simulink model "RHand_20DOF_Inv"  (R2020b)
settings: Solver=ode4  StartTime=0  StopTime=tTimeEnd  FixedStep=iStep  RelTol=1e-20  EnableMultiTasking=on
values from neighbouring files (symbols this model uses):
  g = 9.81    [getStaticTroques.m]    (also in ini_simbody_hand_19DOF.m; setModelParam_BoxSci.m)
  N = 18    [getStaticTroques.m]
undefined symbols (not defined in the file or in its folder): dof_mech_ra_cmc1_ad_ab, dof_mech_ra_cmc1_f_e, dof_mech_ra_dip2_e_f, dof_mech_ra_dip3_e_f, dof_mech_ra_dip4_e_f, dof_mech_ra_dip5_e_f, dof_mech_ra_el_e_f, dof_mech_ra_ip1_f_e, dof_mech_ra_mcp1_f_e, dof_mech_ra_mcp2_e_f, dof_mech_ra_mcp3_e_f, dof_mech_ra_mcp4_e_f, dof_mech_ra_mcp5_e_f, dof_mech_ra_pip2_e_f, dof_mech_ra_pip3_e_f, dof_mech_ra_pip4_e_f, dof_mech_ra_pip5_e_f, dof_mech_ra_wr_ad_ab, dof_mech_ra_wr_e_f, dof_mech_ra_wr_s_p, ic_ra_cmc1_ad_ab, ic_ra_cmc1_f_e, ic_ra_dip2_e_f, ic_ra_dip3_e_f, ic_ra_dip4_e_f, ic_ra_dip5_e_f, ic_ra_el_e_f, ic_ra_ip1_f_e, ic_ra_mcp1_f_e, ic_ra_mcp2_e_f, ic_ra_mcp3_e_f, ic_ra_mcp4_e_f, ic_ra_mcp5_e_f, ic_ra_pip2_e_f, ic_ra_pip3_e_f, ic_ra_pip4_e_f, ic_ra_pip5_e_f, ic_ra_wr_ad_ab, ic_ra_wr_e_f, ic_ra_wr_s_p, nScale, range_ra_cmc1_ad_ab, range_ra_cmc1_f_e, range_ra_dip2_e_f, range_ra_dip3_e_f, range_ra_dip4_e_f, range_ra_dip5_e_f, range_ra_el_e_f, range_ra_ip1_f_e, range_ra_mcp1_f_e, range_ra_mcp2_e_f, range_ra_mcp3_e_f, range_ra_mcp4_e_f, range_ra_mcp5_e_f, range_ra_pip2_e_f, range_ra_pip3_e_f, range_ra_pip4_e_f, range_ra_pip5_e_f, range_ra_wr_ad_ab, range_ra_wr_e_f ... (+4)
libraries: sm_lib x116, nesl_utility x41
(part 1 of 4)
settings Model: Creator=valeriya  LastModifiedBy=matthewyough
settings SolverCC: ShapePreserveControl=EnableAll  ZeroCrossControl=EnableAll  ZeroCrossAlgorithm=Adaptive  AutoInsertRateTranBlk=on
settings DataIOCC: SaveFormat=Array  SaveOutput=off  SignalLogging=off  DSMLogging=off  SaveTime=off  ReturnWorkspaceOutputs=off
settings OptimizationCC: LifeSpan=inf
settings DebuggingCC: InheritedTsInSrcMsg=none  SFUnexpectedBacktrackingDiag=warning  SFNoUnconditionalDefaultTransitionDiag=warning  SFExecutionAtInitializationDiag=none  ArithmeticOperatorsInVariantConditions=warning
settings HardwareCC: ProdBitPerPointer=32  ProdBitPerSizeT=32  ProdBitPerPtrDiffT=32  ProdLargestAtomicFloat=None  ProdIntDivRoundTo=Undefined  ProdEndianess=Unspecified  ProdWordSize=32  ProdHWDeviceType=32-bit Generic
settings ModelReferenceCC: PropagateSignalLabelsOutOfModel=off
settings SFSimCC: SimUseLocalCustomCode=off  CustomCodeUndefinedFunction=UseInterfaceOnly
settings RTWCC: RTWUseLocalCustomCode=off
settings CodeAppCC: StateflowObjectComments=on
settings GRTTargetCC: TargetLangStandard=C89/C90 (ANSI)
settings ConfigComp: CovMetricSettings=dw  CovSaveCumulativeToWorkspaceVar=on  CovSaveSingleToWorkspaceVar=on  CovExternalEMLEnable=off
settings SimscapeCC: SimscapeNormalizeSystem=off  SimscapeLogLimitData=off  SimscapeLogDataHistory=10000
settings ConfigurationSet: Description=SimMechanics 2G

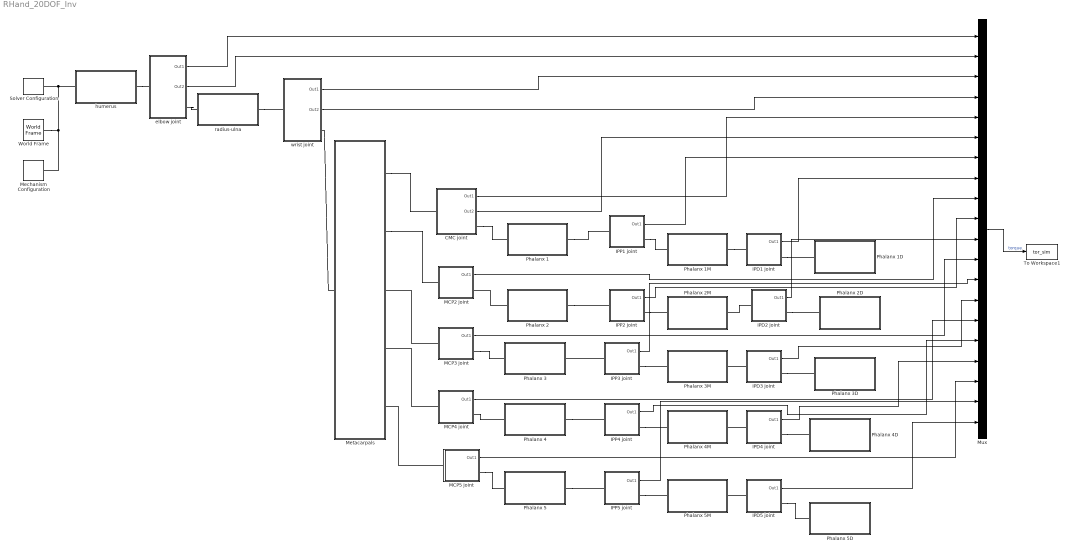
== system RHand_20DOF_Inv ==
  CMC joint : Subsystem
  IPD1 joint : Subsystem
  IPD2 joint : Subsystem
  IPD3 joint : Subsystem
  IPD4 joint : Subsystem
  IPD5 joint : Subsystem
  IPP1 joint : Subsystem
  IPP2 joint : Subsystem
  IPP3 joint : Subsystem
  IPP4 joint : Subsystem
  IPP5 joint : Subsystem
  MCP2 joint : Subsystem
  MCP3 joint : Subsystem
  MCP4 joint : Subsystem
  MCP5 joint : Subsystem
  Mechanism Configuration : sm_lib/Utilities/Mechanism Configuration  UniformGravity=Constant  GravityVector=[0 g 0]  GravityVectorUnits=m/s^2  GravityUnits=m/s^2  LinearizationDelta=0.000001  JointModeTransitionNonlinearIterations=2
  Metacarpals : Subsystem  mask{L=nScale.MC(1), W=nScale.MC(2), T=nScale.MC(3), CM=nScale.MC(4), M=nScale.MC(5)}
      mask prompts: L "Length (m)"; W "Width (m)"; T "Thickness (m)"; CM "Center of mass (m)"; M "Mass (kg)"
  Mux : Mux  Inputs=20
  Phalanx 1 : Subsystem  mask{L=nScale.P1(1), R=nScale.P1(2), CM=nScale.P1(4), M=nScale.P1(5)}
      mask prompts: L "Segment length (m)"; R "Segment radius (m)"; CM "Distance to the center of mass (m)"; M "Segment mass (kg)"
  Phalanx 1D : Subsystem  mask{L=nScale.P1D(1), R=nScale.P1D(2), CM=nScale.P1D(4), M=nScale.P1D(5)}
      mask prompts: L "Segment length (m)"; R "Segment radius (m)"; CM "Distance to the center of mass (m)"; M "Segment mass (kg)"
  Phalanx 1M : Subsystem  mask{L=nScale.P1M(1), R=nScale.P1M(2), CM=nScale.P1M(4), M=nScale.P1M(5)}
      mask prompts: L "Segment length (m)"; R "Segment radius (m)"; CM "Distance to the center of mass (m)"; M "Segment mass (kg)"
  Phalanx 2 : Subsystem  mask{L=nScale.P2(1), R=nScale.P2(2), CM=nScale.P2(4), M=nScale.P2(5)}
      mask prompts: L "Segment length (m)"; R "Segment radius (m)"; CM "Distance to the center of mass (m)"; M "Segment mass (kg)"
  Phalanx 2D : Subsystem  mask{L=nScale.P2D(1), R=nScale.P2D(2), CM=nScale.P2D(4), M=nScale.P2D(5)}
      mask prompts: L "Segment length (m)"; R "Segment radius (m)"; CM "Distance to the center of mass (m)"; M "Segment mass (kg)"
  Phalanx 2M : Subsystem  mask{L=nScale.P2M(1), R=nScale.P2M(2), CM=nScale.P2M(4), M=nScale.P2M(5)}
      mask prompts: L "Segment length (m)"; R "Segment radius (m)"; CM "Distance to the center of mass (m)"; M "Segment mass (kg)"
  Phalanx 3 : Subsystem  mask{L=nScale.P3(1), R=nScale.P3(2), CM=nScale.P3(4), M=nScale.P3(5)}
      mask prompts: L "Segment length (m)"; R "Segment radius (m)"; CM "Distance to the center of mass (m)"; M "Segment mass (kg)"
  Phalanx 3D : Subsystem  mask{L=nScale.P3D(1), R=nScale.P3D(2), CM=nScale.P3D(4), M=nScale.P3D(5)}
      mask prompts: L "Segment length (m)"; R "Segment radius (m)"; CM "Distance to the center of mass (m)"; M "Segment mass (kg)"
  Phalanx 3M : Subsystem  mask{L=nScale.P3M(1), R=nScale.P3M(2), CM=nScale.P3M(4), M=nScale.P3M(5)}
      mask prompts: L "Segment length (m)"; R "Segment radius (m)"; CM "Distance to the center of mass (m)"; M "Segment mass (kg)"
  Phalanx 4 : Subsystem  mask{L=nScale.P4(1), R=nScale.P4(2), CM=nScale.P4(4), M=nScale.P4(5)}
      mask prompts: L "Segment length (m)"; R "Segment radius (m)"; CM "Distance to the center of mass (m)"; M "Segment mass (kg)"
  Phalanx 4D : Subsystem  mask{L=nScale.P4D(1), R=nScale.P4D(2), CM=nScale.P4D(4), M=nScale.P4D(5)}
      mask prompts: L "Segment length (m)"; R "Segment radius (m)"; CM "Distance to the center of mass (m)"; M "Segment mass (kg)"
  Phalanx 4M : Subsystem  mask{L=nScale.P4M(1), R=nScale.P4M(2), CM=nScale.P4M(4), M=nScale.P4M(5)}
      mask prompts: L "Segment length (m)"; R "Segment radius (m)"; CM "Distance to the center of mass (m)"; M "Segment mass (kg)"
  Phalanx 5 : Subsystem  mask{L=nScale.P5(1), R=nScale.P5(2), CM=nScale.P5(4), M=nScale.P5(5)}
      mask prompts: L "Segment length (m)"; R "Segment radius (m)"; CM "Distance to the center of mass (m)"; M "Segment mass (kg)"
  Phalanx 5D : Subsystem  mask{L=nScale.P5D(1), R=nScale.P5D(2), CM=nScale.P5D(4), M=nScale.P5D(5)}
      mask prompts: L "Segment length (m)"; R "Segment radius (m)"; CM "Distance to the center of mass (m)"; M "Segment mass (kg)"
  Phalanx 5M : Subsystem  mask{L=nScale.P5M(1), R=nScale.P5M(2), CM=nScale.P5M(4), M=nScale.P5M(5)}
      mask prompts: L "Segment length (m)"; R "Segment radius (m)"; CM "Distance to the center of mass (m)"; M "Segment mass (kg)"
  Solver Configuration : nesl_utility/Solver Configuration  PhysicalDomain=network_engine_domain  SubClassName=solver  LeftPortType=input  RightPortType=generic  Tones=[]  Harmonics=[]  SimulateNoise=off  Profile=off  UseLocalSampling=off  EnableSwitchedLinearOptims=on  FrequencyDomain=off  UseCCode=off  RelTol=0.001  AbsTol=1e-06  MinStep=1e-09  ToWorkspace=off  RevertToSquareIcSolve=off  NumHomotopyIterations=100  PhasorMode=off  PhasorModeNumHarmonics=1  DoDC=on  ResidualTolerance=1e-48  UseLocalSolver=off  LocalSolverChoice=NE_BACKWARD_EULER_ADVANCER  LocalSolverSampleTime=iStep  DoFixedCost=off  MaxNonlinIter=3  MaxModeIter=2  ComputeImpulses=off  ImpulseIterations=2  LinearAlgebra=Full  EquationFormulation=NE_TIME_EF  DelaysMemoryBudget=1024  AutomaticFiltering=off  FilteringTimeConstant=0.01  PartitionStorageMethod=AS_NEEDED  PartitionMemoryBudget=1024  PartitionMethod=FAST
  To Workspace1 : ToWorkspace  VariableName=tor_sim  SaveFormat=Structure With Time  SampleTime=-1
  World Frame : sm_lib/Frames and Transforms/World Frame
  elbow joint : Subsystem
  humerus : Subsystem  mask{L=nScale.H(1), R=nScale.H(2), CM=nScale.H(4), M=nScale.H(5)}
      mask prompts: L "Segment length (m)"; R "Segment radius (m)"; CM "Distance to the center of mass (m)"; M "Segment mass (kg)"
  radius-ulna : Subsystem  mask{L=nScale.RU(1), R=nScale.RU(2), CM=nScale.RU(4), M=nScale.RU(5)}
      mask prompts: L "Segment length (m)"; R "Segment radius (m)"; CM "Distance to the center of mass (m)"; M "Segment mass (kg)"
  wrist joint : Subsystem
  wires:
  Mux/1 -> To Workspace1/1  "torque"
  elbow joint/1(Out1) -> Mux/1
  elbow joint/2(Out2) -> Mux/2
  wrist joint/2(Out2) -> Mux/4
  wrist joint/1(Out1) -> Mux/3
  CMC joint/1(Out1) -> Mux/5
  CMC joint/2(Out2) -> Mux/6
  IPP1 joint/1(Out1) -> Mux/7
  IPD1 joint/1(Out1) -> Mux/8
  IPD5 joint/1(Out1) -> Mux/20
  IPD2 joint/1(Out1) -> Mux/11
  IPP2 joint/1(Out1) -> Mux/10
  IPD3 joint/1(Out1) -> Mux/14
  IPD4 joint/1(Out1) -> Mux/17
  IPP5 joint/1(Out1) -> Mux/19
  IPP4 joint/1(Out1) -> Mux/16
  MCP5 joint/1(Out1) -> Mux/18
  MCP2 joint/1(Out1) -> Mux/9
  IPP3 joint/1(Out1) -> Mux/13
  MCP3 joint/1(Out1) -> Mux/12
  MCP4 joint/1(Out1) -> Mux/15
  connections:
  World Frame/RConn1 -- Solver Configuration/RConn1 -- humerus/LConn1 -- Mechanism Configuration/RConn1
  Metacarpals/LConn1 -- wrist joint/RConn1
  radius-ulna/RConn1 -- wrist joint/LConn1
  humerus/RConn1 -- elbow joint/LConn1
  elbow joint/RConn1 -- radius-ulna/LConn1
  Metacarpals/RConn1 -- CMC joint/LConn1
  CMC joint/RConn1 -- Phalanx 1/LConn1
  IPP1 joint/RConn1 -- Phalanx 1M/LConn1
  Phalanx 1/RConn1 -- IPP1 joint/LConn1
  IPD1 joint/RConn1 -- Phalanx 1D/LConn1
  Phalanx 1M/RConn1 -- IPD1 joint/LConn1
  IPP4 joint/RConn1 -- Phalanx 4M/LConn1
  Metacarpals/RConn2 -- MCP2 joint/LConn1
  Phalanx 4/RConn1 -- IPP4 joint/LConn1
  IPD4 joint/RConn1 -- Phalanx 4D/LConn1
  MCP4 joint/RConn1 -- Phalanx 4/LConn1
  IPD3 joint/LConn1 -- Phalanx 3M/RConn1
  Phalanx 2/RConn1 -- IPP2 joint/LConn1
  IPP3 joint/RConn1 -- Phalanx 3M/LConn1
  Phalanx 5/RConn1 -- IPP5 joint/LConn1
  IPD5 joint/LConn1 -- Phalanx 5M/RConn1
  IPD4 joint/LConn1 -- Phalanx 4M/RConn1
  IPP2 joint/RConn1 -- Phalanx 2M/LConn1
  MCP5 joint/RConn1 -- Phalanx 5/LConn1
  IPP3 joint/LConn1 -- Phalanx 3/RConn1
  IPD5 joint/RConn1 -- Phalanx 5D/LConn1
  Phalanx 2/LConn1 -- MCP2 joint/RConn1
  IPD2 joint/RConn1 -- Phalanx 2D/LConn1
  IPP5 joint/RConn1 -- Phalanx 5M/LConn1
  IPD2 joint/LConn1 -- Phalanx 2M/RConn1
  MCP3 joint/RConn1 -- Phalanx 3/LConn1
  IPD3 joint/RConn1 -- Phalanx 3D/LConn1
  MCP3 joint/LConn1 -- Metacarpals/RConn3
  MCP4 joint/LConn1 -- Metacarpals/RConn4
  MCP5 joint/LConn1 -- Metacarpals/RConn5

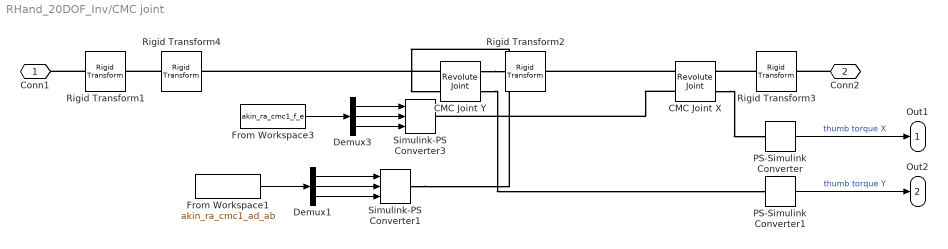
== system RHand_20DOF_Inv/CMC joint ==
  CMC Joint X : sm_lib/Joints/Revolute Joint  JointMode=Normal  SenseConstraintForce=off  SenseConstraintForceX=off  SenseConstraintForceY=off  SenseConstraintForceZ=off  SenseConstraintTorque=off  SenseConstraintTorqueX=off  SenseConstraintTorqueY=off  SenseConstraintTorqueZ=off  SenseTotalForce=off  SenseTotalForceX=off  SenseTotalForceY=off  SenseTotalForceZ=off  SenseTotalTorque=off  SenseTotalTorqueX=off  SenseTotalTorqueY=off  SenseTotalTorqueZ=off  CompositeWrenchDir=FollowerOnBase  CompositeWrenchFrame=BaseFrame  EquilibriumPosition=dof_mech_ra_cmc1_f_e(1)  EquilibriumPositionUnits=rad  SpringStiffness=dof_mech_ra_cmc1_f_e(2)  SpringStiffnessUnits=N*m/rad  DampingCoefficient=dof_mech_ra_cmc1_f_e(3)  DampingCoefficientUnits=N*m/(rad/s)  TorqueActuationMode=ComputedTorque  MotionActuationMode=InputMotion  SensePosition=off  SenseVelocity=off  SenseAcceleration=off  SenseTorqueForce=on  SenseLowerLimitTorqueForce=off  SenseUpperLimitTorqueForce=off  LowerLimitSpecify=on  LowerLimitBound=range_ra_cmc1_f_e(1)  LowerLimitBoundUnits=deg  LowerLimitStiffness=1e4  LowerLimitStiffnessUnits=N*m/deg  LowerLimitDamping=10  LowerLimitDampingUnits=N*m/(deg/s)  LowerLimitTransitionRegionWidth=0.1  LowerLimitTransitionRegionWidthUnits=deg  UpperLimitSpecify=on  UpperLimitBound=range_ra_cmc1_f_e(2)  UpperLimitBoundUnits=deg  UpperLimitStiffness=1e4  UpperLimitStiffnessUnits=N*m/deg  UpperLimitDamping=10  UpperLimitDampingUnits=N*m/(deg/s)  UpperLimitTransitionRegionWidth=0.1  UpperLimitTransitionRegionWidthUnits=deg  PositionTargetSpecify=off  PositionTargetPriority=High  PositionTargetValue=ic_ra_cmc1_f_e(1)  PositionTargetValueUnits=rad  VelocityTargetSpecify=off  VelocityTargetPriority=High  VelocityTargetValue=ic_ra_cmc1_f_e(2)  VelocityTargetValueUnits=rad/s
  CMC Joint Y : sm_lib/Joints/Revolute Joint  JointMode=Normal  SenseConstraintForce=off  SenseConstraintForceX=off  SenseConstraintForceY=off  SenseConstraintForceZ=off  SenseConstraintTorque=off  SenseConstraintTorqueX=off  SenseConstraintTorqueY=off  SenseConstraintTorqueZ=off  SenseTotalForce=off  SenseTotalForceX=off  SenseTotalForceY=off  SenseTotalForceZ=off  SenseTotalTorque=off  SenseTotalTorqueX=off  SenseTotalTorqueY=off  SenseTotalTorqueZ=off  CompositeWrenchDir=FollowerOnBase  CompositeWrenchFrame=BaseFrame  EquilibriumPosition=dof_mech_ra_cmc1_ad_ab(1)  EquilibriumPositionUnits=rad  SpringStiffness=dof_mech_ra_cmc1_ad_ab(2)  SpringStiffnessUnits=N*m/rad  DampingCoefficient=dof_mech_ra_cmc1_ad_ab(3)  DampingCoefficientUnits=N*m/(rad/s)  TorqueActuationMode=ComputedTorque  MotionActuationMode=InputMotion  SensePosition=off  SenseVelocity=off  SenseAcceleration=off  SenseTorqueForce=on  SenseLowerLimitTorqueForce=off  SenseUpperLimitTorqueForce=off  LowerLimitSpecify=on  LowerLimitBound=range_ra_cmc1_ad_ab(1)  LowerLimitBoundUnits=deg  LowerLimitStiffness=1e4  LowerLimitStiffnessUnits=N*m/deg  LowerLimitDamping=10  LowerLimitDampingUnits=N*m/(deg/s)  LowerLimitTransitionRegionWidth=0.1  LowerLimitTransitionRegionWidthUnits=deg  UpperLimitSpecify=on  UpperLimitBound=range_ra_cmc1_ad_ab(2)  UpperLimitBoundUnits=deg  UpperLimitStiffness=1e4  UpperLimitStiffnessUnits=N*m/deg  UpperLimitDamping=10  UpperLimitDampingUnits=N*m/(deg/s)  UpperLimitTransitionRegionWidth=0.1  UpperLimitTransitionRegionWidthUnits=deg  PositionTargetSpecify=off  PositionTargetPriority=High  PositionTargetValue=ic_ra_cmc1_ad_ab(1)  PositionTargetValueUnits=rad  VelocityTargetSpecify=off  VelocityTargetPriority=High  VelocityTargetValue=ic_ra_cmc1_ad_ab(2)  VelocityTargetValueUnits=rad/s
  Demux1 : Demux  Outputs=3
  Demux3 : Demux  Outputs=3
  From Workspace1 : FromWorkspace  VariableName=akin_ra_cmc1_ad_ab  SampleTime=-1  OutputAfterFinalValue=Holding final value
  From Workspace3 : FromWorkspace  VariableName=akin_ra_cmc1_f_e  SampleTime=-1  OutputAfterFinalValue=Holding final value
  PS-Simulink Converter : nesl_utility/PS-Simulink Converter  PhysicalDomain=network_engine_domain  SubClassName=ps_output  LeftPortType=input  RightPortType=output  PseudoPeriodic=off  Frequencies=[]  Unit=N*m  AffineConversion=off
  PS-Simulink Converter1 : nesl_utility/PS-Simulink Converter  PhysicalDomain=network_engine_domain  SubClassName=ps_output  LeftPortType=input  RightPortType=output  PseudoPeriodic=off  Frequencies=[]  Unit=N*m  AffineConversion=off
  Rigid Transform1 : sm_lib/Frames and Transforms/Rigid Transform  TranslationMethod=None  TranslationStandardOffset=0  TranslationLengthUnit=m  TranslationStandardAxis=+Z  TranslationCartesianOffset=[0 0 0]  TranslationROffset=0  TranslationROffsetUnits=m  TranslationZOffset=0  TranslationZOffsetUnits=m  TranslationThetaOffset=0  TranslationThetaOffsetUnits=deg  RotationMethod=StandardAxis  RotationAngleUnits=deg  RotationStandardAxis=-X  RotationAngle=180  RotationArbitraryAxis=[0 0 1]  FollAlignAxisA=+X  BaseAlignAxisA=+Y  FollAlignAxisB=+Y  BaseAlignAxisB=+Z  RotationSequenceAxes=FollowerAxes  RotationSequence=XYX  RotationSequenceAngles=[0 0 0]  RotationSequenceAnglesUnits=deg  RotationMatrix=[1 0 0; 0 1 0; 0 0 1]
  Rigid Transform2 : sm_lib/Frames and Transforms/Rigid Transform  TranslationMethod=None  TranslationStandardOffset=0  TranslationLengthUnit=m  TranslationStandardAxis=+Z  TranslationCartesianOffset=[0 0 0]  TranslationROffset=0  TranslationROffsetUnits=m  TranslationZOffset=0  TranslationZOffsetUnits=m  TranslationThetaOffset=0  TranslationThetaOffsetUnits=deg  RotationMethod=StandardAxis  RotationAngleUnits=deg  RotationStandardAxis=+Y  RotationAngle=90  RotationArbitraryAxis=[0 0 1]  FollAlignAxisA=+X  BaseAlignAxisA=+Y  FollAlignAxisB=+Y  BaseAlignAxisB=+Z  RotationSequenceAxes=FollowerAxes  RotationSequence=XYX  RotationSequenceAngles=[0 0 0]  RotationSequenceAnglesUnits=deg  RotationMatrix=[1 0 0; 0 1 0; 0 0 1]
  Rigid Transform3 : sm_lib/Frames and Transforms/Rigid Transform  TranslationMethod=None  TranslationStandardOffset=0  TranslationLengthUnit=m  TranslationStandardAxis=+Z  TranslationCartesianOffset=[0 0 0]  TranslationROffset=0  TranslationROffsetUnits=m  TranslationZOffset=0  TranslationZOffsetUnits=m  TranslationThetaOffset=0  TranslationThetaOffsetUnits=deg  RotationMethod=StandardAxis  RotationAngleUnits=deg  RotationStandardAxis=+X  RotationAngle=90  RotationArbitraryAxis=[0 0 1]  FollAlignAxisA=+X  BaseAlignAxisA=+Y  FollAlignAxisB=+Y  BaseAlignAxisB=+Z  RotationSequenceAxes=FollowerAxes  RotationSequence=XYX  RotationSequenceAngles=[0 0 0]  RotationSequenceAnglesUnits=deg  RotationMatrix=[1 0 0; 0 1 0; 0 0 1]
  Rigid Transform4 : sm_lib/Frames and Transforms/Rigid Transform  TranslationMethod=None  TranslationStandardOffset=0  TranslationLengthUnit=m  TranslationStandardAxis=+Z  TranslationCartesianOffset=[0 0 0]  TranslationROffset=0  TranslationROffsetUnits=m  TranslationZOffset=0  TranslationZOffsetUnits=m  TranslationThetaOffset=0  TranslationThetaOffsetUnits=deg  RotationMethod=StandardAxis  RotationAngleUnits=deg  RotationStandardAxis=+Y  RotationAngle=90  RotationArbitraryAxis=[0 0 1]  FollAlignAxisA=+X  BaseAlignAxisA=+Y  FollAlignAxisB=+Y  BaseAlignAxisB=+Z  RotationSequenceAxes=FollowerAxes  RotationSequence=XYX  RotationSequenceAngles=[0 0 0]  RotationSequenceAnglesUnits=deg  RotationMatrix=[1 0 0; 0 1 0; 0 0 1]
  Simulink-PS Converter1 : nesl_utility/Simulink-PS Converter  PhysicalDomain=network_engine_domain  SubClassName=ps_input  LeftPortType=input  RightPortType=output  PseudoPeriodic=off  Frequencies=[]  NoiseDistribution=none  NoiseParameters=[]  Unit=rad  AffineConversion=on  FilteringAndDerivatives=provide  SimscapeFilterOrder=2  InputFilterTimeConstant=0.001  UdotUserProvided=2
  Simulink-PS Converter3 : nesl_utility/Simulink-PS Converter  PhysicalDomain=network_engine_domain  SubClassName=ps_input  LeftPortType=input  RightPortType=output  PseudoPeriodic=off  Frequencies=[]  NoiseDistribution=none  NoiseParameters=[]  Unit=rad  AffineConversion=on  FilteringAndDerivatives=provide  SimscapeFilterOrder=2  InputFilterTimeConstant=0.001  UdotUserProvided=2
  Conn1 : PMIOPort  Side=Left
  Conn2 : PMIOPort  Port=2  Side=Right
  Out1 : Outport  VectorParamsAs1DForOutWhenUnconnected=off
  Out2 : Outport  Port=2  VectorParamsAs1DForOutWhenUnconnected=off
  wires:
  Demux3/1 -> Simulink-PS Converter3/1
  From Workspace3/1 -> Demux3/1
  Demux3/3 -> Simulink-PS Converter3/3
  Demux3/2 -> Simulink-PS Converter3/2
  Demux1/1 -> Simulink-PS Converter1/1
  From Workspace1/1 -> Demux1/1
  Demux1/3 -> Simulink-PS Converter1/3
  Demux1/2 -> Simulink-PS Converter1/2
  PS-Simulink Converter/1 -> Out1/1  "thumb torque X"
  PS-Simulink Converter1/1 -> Out2/1  "thumb torque Y"
  connections:
  CMC Joint X/LConn2 -- Simulink-PS Converter3/RConn1
  CMC Joint X/RConn2 -- PS-Simulink Converter/LConn1
  Rigid Transform1/LConn1 -- Conn1/RConn1
  CMC Joint Y/LConn1 -- Rigid Transform4/RConn1
  Simulink-PS Converter1/RConn1 -- CMC Joint Y/LConn2
  CMC Joint Y/RConn2 -- PS-Simulink Converter1/LConn1
  CMC Joint Y/RConn1 -- Rigid Transform2/LConn1
  CMC Joint X/LConn1 -- Rigid Transform2/RConn1
  Conn2/RConn1 -- Rigid Transform3/RConn1
  Rigid Transform4/LConn1 -- Rigid Transform1/RConn1
  Rigid Transform3/LConn1 -- CMC Joint X/RConn1

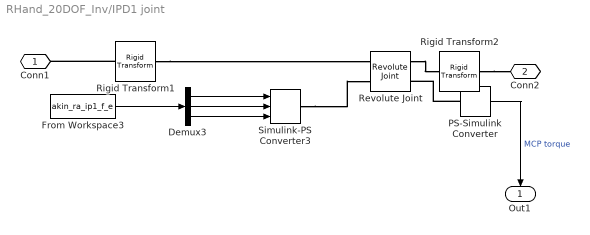
== system RHand_20DOF_Inv/IPD1 joint ==
  Demux3 : Demux  Outputs=3
  From Workspace3 : FromWorkspace  VariableName=akin_ra_ip1_f_e  SampleTime=-1  OutputAfterFinalValue=Holding final value
  PS-Simulink Converter : nesl_utility/PS-Simulink Converter  PhysicalDomain=network_engine_domain  SubClassName=ps_output  LeftPortType=input  RightPortType=output  PseudoPeriodic=off  Frequencies=[]  Unit=N*m  AffineConversion=off
  Revolute Joint : sm_lib/Joints/Revolute Joint  JointMode=Normal  SenseConstraintForce=off  SenseConstraintForceX=off  SenseConstraintForceY=off  SenseConstraintForceZ=off  SenseConstraintTorque=off  SenseConstraintTorqueX=off  SenseConstraintTorqueY=off  SenseConstraintTorqueZ=off  SenseTotalForce=off  SenseTotalForceX=off  SenseTotalForceY=off  SenseTotalForceZ=off  SenseTotalTorque=off  SenseTotalTorqueX=off  SenseTotalTorqueY=off  SenseTotalTorqueZ=off  CompositeWrenchDir=FollowerOnBase  CompositeWrenchFrame=BaseFrame  EquilibriumPosition=dof_mech_ra_ip1_f_e(1)  EquilibriumPositionUnits=rad  SpringStiffness=dof_mech_ra_ip1_f_e(2)  SpringStiffnessUnits=N*m/rad  DampingCoefficient=dof_mech_ra_ip1_f_e(3)  DampingCoefficientUnits=N*m/(rad/s)  TorqueActuationMode=ComputedTorque  MotionActuationMode=InputMotion  SensePosition=off  SenseVelocity=off  SenseAcceleration=off  SenseTorqueForce=on  SenseLowerLimitTorqueForce=off  SenseUpperLimitTorqueForce=off  LowerLimitSpecify=on  LowerLimitBound=range_ra_ip1_f_e(1)  LowerLimitBoundUnits=deg  LowerLimitStiffness=1e4  LowerLimitStiffnessUnits=N*m/deg  LowerLimitDamping=10  LowerLimitDampingUnits=N*m/(deg/s)  LowerLimitTransitionRegionWidth=0.1  LowerLimitTransitionRegionWidthUnits=deg  UpperLimitSpecify=on  UpperLimitBound=range_ra_ip1_f_e(2)  UpperLimitBoundUnits=deg  UpperLimitStiffness=1e4  UpperLimitStiffnessUnits=N*m/deg  UpperLimitDamping=10  UpperLimitDampingUnits=N*m/(deg/s)  UpperLimitTransitionRegionWidth=0.1  UpperLimitTransitionRegionWidthUnits=deg  PositionTargetSpecify=off  PositionTargetPriority=High  PositionTargetValue=ic_ra_ip1_f_e(1)  PositionTargetValueUnits=rad  VelocityTargetSpecify=off  VelocityTargetPriority=High  VelocityTargetValue=ic_ra_ip1_f_e(2)  VelocityTargetValueUnits=rad/s
  Rigid Transform1 : sm_lib/Frames and Transforms/Rigid Transform  TranslationMethod=None  TranslationStandardOffset=0  TranslationLengthUnit=m  TranslationStandardAxis=+Z  TranslationCartesianOffset=[0 0 0]  TranslationROffset=0  TranslationROffsetUnits=m  TranslationZOffset=0  TranslationZOffsetUnits=m  TranslationThetaOffset=0  TranslationThetaOffsetUnits=deg  RotationMethod=StandardAxis  RotationAngleUnits=deg  RotationStandardAxis=-X  RotationAngle=90  RotationArbitraryAxis=[0 0 1]  FollAlignAxisA=+X  BaseAlignAxisA=+Y  FollAlignAxisB=+Y  BaseAlignAxisB=+Z  RotationSequenceAxes=FollowerAxes  RotationSequence=XYX  RotationSequenceAngles=[0 0 0]  RotationSequenceAnglesUnits=deg  RotationMatrix=[1 0 0; 0 1 0; 0 0 1]
  Rigid Transform2 : sm_lib/Frames and Transforms/Rigid Transform  TranslationMethod=None  TranslationStandardOffset=0  TranslationLengthUnit=m  TranslationStandardAxis=+Z  TranslationCartesianOffset=[0 0 0]  TranslationROffset=0  TranslationROffsetUnits=m  TranslationZOffset=0  TranslationZOffsetUnits=m  TranslationThetaOffset=0  TranslationThetaOffsetUnits=deg  RotationMethod=StandardAxis  RotationAngleUnits=deg  RotationStandardAxis=+X  RotationAngle=90  RotationArbitraryAxis=[0 0 1]  FollAlignAxisA=+X  BaseAlignAxisA=+Y  FollAlignAxisB=+Y  BaseAlignAxisB=+Z  RotationSequenceAxes=FollowerAxes  RotationSequence=XYX  RotationSequenceAngles=[0 0 0]  RotationSequenceAnglesUnits=deg  RotationMatrix=[1 0 0; 0 1 0; 0 0 1]
  Simulink-PS Converter3 : nesl_utility/Simulink-PS Converter  PhysicalDomain=network_engine_domain  SubClassName=ps_input  LeftPortType=input  RightPortType=output  PseudoPeriodic=off  Frequencies=[]  NoiseDistribution=none  NoiseParameters=[]  Unit=rad  AffineConversion=on  FilteringAndDerivatives=provide  SimscapeFilterOrder=2  InputFilterTimeConstant=0.001  UdotUserProvided=2
  Conn1 : PMIOPort  Side=Left
  Conn2 : PMIOPort  Port=2  Side=Right
  Out1 : Outport  VectorParamsAs1DForOutWhenUnconnected=off
  wires:
  Demux3/1 -> Simulink-PS Converter3/1
  From Workspace3/1 -> Demux3/1
  Demux3/3 -> Simulink-PS Converter3/3
  PS-Simulink Converter/1 -> Out1/1  "MCP torque"
  Demux3/2 -> Simulink-PS Converter3/2
  connections:
  Simulink-PS Converter3/RConn1 -- Revolute Joint/LConn2
  PS-Simulink Converter/LConn1 -- Revolute Joint/RConn2
  Revolute Joint/RConn1 -- Rigid Transform2/LConn1
  Rigid Transform1/LConn1 -- Conn1/RConn1
  Rigid Transform1/RConn1 -- Revolute Joint/LConn1
  Rigid Transform2/RConn1 -- Conn2/RConn1

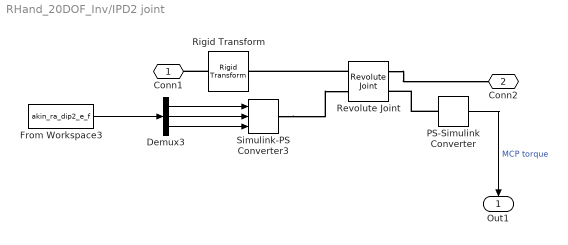
== system RHand_20DOF_Inv/IPD2 joint ==
  Demux3 : Demux  Outputs=3
  From Workspace3 : FromWorkspace  VariableName=akin_ra_dip2_e_f  SampleTime=-1  OutputAfterFinalValue=Holding final value
  PS-Simulink Converter : nesl_utility/PS-Simulink Converter  PhysicalDomain=network_engine_domain  SubClassName=ps_output  LeftPortType=input  RightPortType=output  PseudoPeriodic=off  Frequencies=[]  Unit=N*m  AffineConversion=off
  Revolute Joint : sm_lib/Joints/Revolute Joint  JointMode=Normal  SenseConstraintForce=off  SenseConstraintForceX=off  SenseConstraintForceY=off  SenseConstraintForceZ=off  SenseConstraintTorque=off  SenseConstraintTorqueX=off  SenseConstraintTorqueY=off  SenseConstraintTorqueZ=off  SenseTotalForce=off  SenseTotalForceX=off  SenseTotalForceY=off  SenseTotalForceZ=off  SenseTotalTorque=off  SenseTotalTorqueX=off  SenseTotalTorqueY=off  SenseTotalTorqueZ=off  CompositeWrenchDir=FollowerOnBase  CompositeWrenchFrame=BaseFrame  EquilibriumPosition=dof_mech_ra_dip2_e_f(1)  EquilibriumPositionUnits=rad  SpringStiffness=dof_mech_ra_dip2_e_f(2)  SpringStiffnessUnits=N*m/rad  DampingCoefficient=dof_mech_ra_dip2_e_f(3)  DampingCoefficientUnits=N*m/(rad/s)  TorqueActuationMode=ComputedTorque  MotionActuationMode=InputMotion  SensePosition=off  SenseVelocity=off  SenseAcceleration=off  SenseTorqueForce=on  SenseLowerLimitTorqueForce=off  SenseUpperLimitTorqueForce=off  LowerLimitSpecify=on  LowerLimitBound=range_ra_dip2_e_f(1)  LowerLimitBoundUnits=deg  LowerLimitStiffness=1e4  LowerLimitStiffnessUnits=N*m/deg  LowerLimitDamping=10  LowerLimitDampingUnits=N*m/(deg/s)  LowerLimitTransitionRegionWidth=0.1  LowerLimitTransitionRegionWidthUnits=deg  UpperLimitSpecify=on  UpperLimitBound=range_ra_dip2_e_f(2)  UpperLimitBoundUnits=deg  UpperLimitStiffness=1e4  UpperLimitStiffnessUnits=N*m/deg  UpperLimitDamping=10  UpperLimitDampingUnits=N*m/(deg/s)  UpperLimitTransitionRegionWidth=0.1  UpperLimitTransitionRegionWidthUnits=deg  PositionTargetSpecify=off  PositionTargetPriority=High  PositionTargetValue=ic_ra_dip2_e_f(1)  PositionTargetValueUnits=rad  VelocityTargetSpecify=off  VelocityTargetPriority=High  VelocityTargetValue=ic_ra_dip2_e_f(2)  VelocityTargetValueUnits=rad/s
  Rigid Transform : sm_lib/Frames and Transforms/Rigid Transform  TranslationMethod=None  TranslationStandardOffset=0  TranslationLengthUnit=m  TranslationStandardAxis=+Z  TranslationCartesianOffset=[0 0 0]  TranslationROffset=0  TranslationROffsetUnits=m  TranslationZOffset=0  TranslationZOffsetUnits=m  TranslationThetaOffset=0  TranslationThetaOffsetUnits=deg  RotationMethod=StandardAxis  RotationAngleUnits=deg  RotationStandardAxis=-Z  RotationAngle=180  RotationArbitraryAxis=[0 0 1]  FollAlignAxisA=+X  BaseAlignAxisA=+Y  FollAlignAxisB=+Y  BaseAlignAxisB=+Z  RotationSequenceAxes=FollowerAxes  RotationSequence=XYX  RotationSequenceAngles=[0 0 0]  RotationSequenceAnglesUnits=deg  RotationMatrix=[1 0 0; 0 1 0; 0 0 1]
  Simulink-PS Converter3 : nesl_utility/Simulink-PS Converter  PhysicalDomain=network_engine_domain  SubClassName=ps_input  LeftPortType=input  RightPortType=output  PseudoPeriodic=off  Frequencies=[]  NoiseDistribution=none  NoiseParameters=[]  Unit=rad  AffineConversion=on  FilteringAndDerivatives=provide  SimscapeFilterOrder=2  InputFilterTimeConstant=0.001  UdotUserProvided=2
  Conn1 : PMIOPort  Side=Left
  Conn2 : PMIOPort  Port=2  Side=Right
  Out1 : Outport  VectorParamsAs1DForOutWhenUnconnected=off
  wires:
  Demux3/1 -> Simulink-PS Converter3/1
  From Workspace3/1 -> Demux3/1
  Demux3/3 -> Simulink-PS Converter3/3
  PS-Simulink Converter/1 -> Out1/1  "MCP torque"
  Demux3/2 -> Simulink-PS Converter3/2
  connections:
  Simulink-PS Converter3/RConn1 -- Revolute Joint/LConn2
  PS-Simulink Converter/LConn1 -- Revolute Joint/RConn2
  Revolute Joint/RConn1 -- Conn2/RConn1
  Revolute Joint/LConn1 -- Rigid Transform/RConn1
  Rigid Transform/LConn1 -- Conn1/RConn1

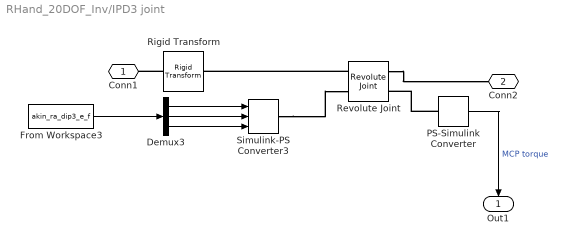
== system RHand_20DOF_Inv/IPD3 joint ==
  Demux3 : Demux  Outputs=3
  From Workspace3 : FromWorkspace  VariableName=akin_ra_dip3_e_f  SampleTime=-1  OutputAfterFinalValue=Holding final value
  PS-Simulink Converter : nesl_utility/PS-Simulink Converter  PhysicalDomain=network_engine_domain  SubClassName=ps_output  LeftPortType=input  RightPortType=output  PseudoPeriodic=off  Frequencies=[]  Unit=N*m  AffineConversion=off
  Revolute Joint : sm_lib/Joints/Revolute Joint  JointMode=Normal  SenseConstraintForce=off  SenseConstraintForceX=off  SenseConstraintForceY=off  SenseConstraintForceZ=off  SenseConstraintTorque=off  SenseConstraintTorqueX=off  SenseConstraintTorqueY=off  SenseConstraintTorqueZ=off  SenseTotalForce=off  SenseTotalForceX=off  SenseTotalForceY=off  SenseTotalForceZ=off  SenseTotalTorque=off  SenseTotalTorqueX=off  SenseTotalTorqueY=off  SenseTotalTorqueZ=off  CompositeWrenchDir=FollowerOnBase  CompositeWrenchFrame=BaseFrame  EquilibriumPosition=dof_mech_ra_dip3_e_f(1)  EquilibriumPositionUnits=rad  SpringStiffness=dof_mech_ra_dip3_e_f(2)  SpringStiffnessUnits=N*m/rad  DampingCoefficient=dof_mech_ra_dip3_e_f(3)  DampingCoefficientUnits=N*m/(rad/s)  TorqueActuationMode=ComputedTorque  MotionActuationMode=InputMotion  SensePosition=off  SenseVelocity=off  SenseAcceleration=off  SenseTorqueForce=on  SenseLowerLimitTorqueForce=off  SenseUpperLimitTorqueForce=off  LowerLimitSpecify=on  LowerLimitBound=range_ra_dip3_e_f(1)  LowerLimitBoundUnits=deg  LowerLimitStiffness=1e4  LowerLimitStiffnessUnits=N*m/deg  LowerLimitDamping=10  LowerLimitDampingUnits=N*m/(deg/s)  LowerLimitTransitionRegionWidth=0.1  LowerLimitTransitionRegionWidthUnits=deg  UpperLimitSpecify=on  UpperLimitBound=range_ra_dip3_e_f(2)  UpperLimitBoundUnits=deg  UpperLimitStiffness=1e4  UpperLimitStiffnessUnits=N*m/deg  UpperLimitDamping=10  UpperLimitDampingUnits=N*m/(deg/s)  UpperLimitTransitionRegionWidth=0.1  UpperLimitTransitionRegionWidthUnits=deg  PositionTargetSpecify=on  PositionTargetPriority=High  PositionTargetValue=ic_ra_dip3_e_f(1)  PositionTargetValueUnits=rad  VelocityTargetSpecify=on  VelocityTargetPriority=High  VelocityTargetValue=ic_ra_dip3_e_f(2)  VelocityTargetValueUnits=rad/s
  Rigid Transform : sm_lib/Frames and Transforms/Rigid Transform  TranslationMethod=None  TranslationStandardOffset=0  TranslationLengthUnit=m  TranslationStandardAxis=+Z  TranslationCartesianOffset=[0 0 0]  TranslationROffset=0  TranslationROffsetUnits=m  TranslationZOffset=0  TranslationZOffsetUnits=m  TranslationThetaOffset=0  TranslationThetaOffsetUnits=deg  RotationMethod=StandardAxis  RotationAngleUnits=deg  RotationStandardAxis=-Z  RotationAngle=180  RotationArbitraryAxis=[0 0 1]  FollAlignAxisA=+X  BaseAlignAxisA=+Y  FollAlignAxisB=+Y  BaseAlignAxisB=+Z  RotationSequenceAxes=FollowerAxes  RotationSequence=XYX  RotationSequenceAngles=[0 0 0]  RotationSequenceAnglesUnits=deg  RotationMatrix=[1 0 0; 0 1 0; 0 0 1]
  Simulink-PS Converter3 : nesl_utility/Simulink-PS Converter  PhysicalDomain=network_engine_domain  SubClassName=ps_input  LeftPortType=input  RightPortType=output  PseudoPeriodic=off  Frequencies=[]  NoiseDistribution=none  NoiseParameters=[]  Unit=rad  AffineConversion=on  FilteringAndDerivatives=provide  SimscapeFilterOrder=2  InputFilterTimeConstant=0.001  UdotUserProvided=2
  Conn1 : PMIOPort  Side=Left
  Conn2 : PMIOPort  Port=2  Side=Right
  Out1 : Outport  VectorParamsAs1DForOutWhenUnconnected=off
  wires:
  Demux3/1 -> Simulink-PS Converter3/1
  From Workspace3/1 -> Demux3/1
  Demux3/3 -> Simulink-PS Converter3/3
  PS-Simulink Converter/1 -> Out1/1  "MCP torque"
  Demux3/2 -> Simulink-PS Converter3/2
  connections:
  Simulink-PS Converter3/RConn1 -- Revolute Joint/LConn2
  PS-Simulink Converter/LConn1 -- Revolute Joint/RConn2
  Revolute Joint/RConn1 -- Conn2/RConn1
  Rigid Transform/LConn1 -- Conn1/RConn1
  Revolute Joint/LConn1 -- Rigid Transform/RConn1

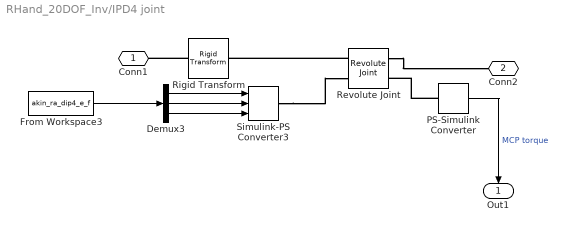
== system RHand_20DOF_Inv/IPD4 joint ==
  Demux3 : Demux  Outputs=3
  From Workspace3 : FromWorkspace  VariableName=akin_ra_dip4_e_f  SampleTime=-1  OutputAfterFinalValue=Holding final value
  PS-Simulink Converter : nesl_utility/PS-Simulink Converter  PhysicalDomain=network_engine_domain  SubClassName=ps_output  LeftPortType=input  RightPortType=output  PseudoPeriodic=off  Frequencies=[]  Unit=N*m  AffineConversion=off
  Revolute Joint : sm_lib/Joints/Revolute Joint  JointMode=Normal  SenseConstraintForce=off  SenseConstraintForceX=off  SenseConstraintForceY=off  SenseConstraintForceZ=off  SenseConstraintTorque=off  SenseConstraintTorqueX=off  SenseConstraintTorqueY=off  SenseConstraintTorqueZ=off  SenseTotalForce=off  SenseTotalForceX=off  SenseTotalForceY=off  SenseTotalForceZ=off  SenseTotalTorque=off  SenseTotalTorqueX=off  SenseTotalTorqueY=off  SenseTotalTorqueZ=off  CompositeWrenchDir=FollowerOnBase  CompositeWrenchFrame=BaseFrame  EquilibriumPosition=dof_mech_ra_dip4_e_f(1)  EquilibriumPositionUnits=rad  SpringStiffness=dof_mech_ra_dip4_e_f(2)  SpringStiffnessUnits=N*m/rad  DampingCoefficient=dof_mech_ra_dip4_e_f(3)  DampingCoefficientUnits=N*m/(rad/s)  TorqueActuationMode=ComputedTorque  MotionActuationMode=InputMotion  SensePosition=off  SenseVelocity=off  SenseAcceleration=off  SenseTorqueForce=on  SenseLowerLimitTorqueForce=off  SenseUpperLimitTorqueForce=off  LowerLimitSpecify=on  LowerLimitBound=range_ra_dip4_e_f(1)  LowerLimitBoundUnits=deg  LowerLimitStiffness=1e4  LowerLimitStiffnessUnits=N*m/deg  LowerLimitDamping=10  LowerLimitDampingUnits=N*m/(deg/s)  LowerLimitTransitionRegionWidth=0.1  LowerLimitTransitionRegionWidthUnits=deg  UpperLimitSpecify=on  UpperLimitBound=range_ra_dip4_e_f(2)  UpperLimitBoundUnits=deg  UpperLimitStiffness=1e4  UpperLimitStiffnessUnits=N*m/deg  UpperLimitDamping=10  UpperLimitDampingUnits=N*m/(deg/s)  UpperLimitTransitionRegionWidth=0.1  UpperLimitTransitionRegionWidthUnits=deg  PositionTargetSpecify=off  PositionTargetPriority=High  PositionTargetValue=ic_ra_dip4_e_f(1)  PositionTargetValueUnits=rad  VelocityTargetSpecify=off  VelocityTargetPriority=High  VelocityTargetValue=ic_ra_dip4_e_f(2)  VelocityTargetValueUnits=rad/s
  Rigid Transform : sm_lib/Frames and Transforms/Rigid Transform  TranslationMethod=None  TranslationStandardOffset=0  TranslationLengthUnit=m  TranslationStandardAxis=+Z  TranslationCartesianOffset=[0 0 0]  TranslationROffset=0  TranslationROffsetUnits=m  TranslationZOffset=0  TranslationZOffsetUnits=m  TranslationThetaOffset=0  TranslationThetaOffsetUnits=deg  RotationMethod=StandardAxis  RotationAngleUnits=deg  RotationStandardAxis=-Z  RotationAngle=180  RotationArbitraryAxis=[0 0 1]  FollAlignAxisA=+X  BaseAlignAxisA=+Y  FollAlignAxisB=+Y  BaseAlignAxisB=+Z  RotationSequenceAxes=FollowerAxes  RotationSequence=XYX  RotationSequenceAngles=[0 0 0]  RotationSequenceAnglesUnits=deg  RotationMatrix=[1 0 0; 0 1 0; 0 0 1]
  Simulink-PS Converter3 : nesl_utility/Simulink-PS Converter  PhysicalDomain=network_engine_domain  SubClassName=ps_input  LeftPortType=input  RightPortType=output  PseudoPeriodic=off  Frequencies=[]  NoiseDistribution=none  NoiseParameters=[]  Unit=rad  AffineConversion=on  FilteringAndDerivatives=provide  SimscapeFilterOrder=2  InputFilterTimeConstant=0.001  UdotUserProvided=2
  Conn1 : PMIOPort  Side=Left
  Conn2 : PMIOPort  Port=2  Side=Right
  Out1 : Outport  VectorParamsAs1DForOutWhenUnconnected=off
  wires:
  Demux3/1 -> Simulink-PS Converter3/1
  From Workspace3/1 -> Demux3/1
  Demux3/3 -> Simulink-PS Converter3/3
  PS-Simulink Converter/1 -> Out1/1  "MCP torque"
  Demux3/2 -> Simulink-PS Converter3/2
  connections:
  Simulink-PS Converter3/RConn1 -- Revolute Joint/LConn2
  PS-Simulink Converter/LConn1 -- Revolute Joint/RConn2
  Revolute Joint/RConn1 -- Conn2/RConn1
  Rigid Transform/LConn1 -- Conn1/RConn1
  Revolute Joint/LConn1 -- Rigid Transform/RConn1

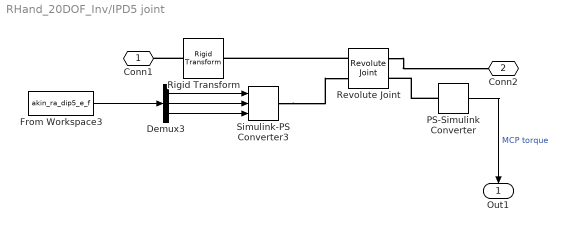
== system RHand_20DOF_Inv/IPD5 joint ==
  Demux3 : Demux  Outputs=3
  From Workspace3 : FromWorkspace  VariableName=akin_ra_dip5_e_f  SampleTime=-1  OutputAfterFinalValue=Holding final value
  PS-Simulink Converter : nesl_utility/PS-Simulink Converter  PhysicalDomain=network_engine_domain  SubClassName=ps_output  LeftPortType=input  RightPortType=output  PseudoPeriodic=off  Frequencies=[]  Unit=N*m  AffineConversion=off
  Revolute Joint : sm_lib/Joints/Revolute Joint  JointMode=Normal  SenseConstraintForce=off  SenseConstraintForceX=off  SenseConstraintForceY=off  SenseConstraintForceZ=off  SenseConstraintTorque=off  SenseConstraintTorqueX=off  SenseConstraintTorqueY=off  SenseConstraintTorqueZ=off  SenseTotalForce=off  SenseTotalForceX=off  SenseTotalForceY=off  SenseTotalForceZ=off  SenseTotalTorque=off  SenseTotalTorqueX=off  SenseTotalTorqueY=off  SenseTotalTorqueZ=off  CompositeWrenchDir=FollowerOnBase  CompositeWrenchFrame=BaseFrame  EquilibriumPosition=dof_mech_ra_dip5_e_f(1)  EquilibriumPositionUnits=rad  SpringStiffness=dof_mech_ra_dip5_e_f(2)  SpringStiffnessUnits=N*m/rad  DampingCoefficient=dof_mech_ra_dip5_e_f(3)  DampingCoefficientUnits=N*m/(rad/s)  TorqueActuationMode=ComputedTorque  MotionActuationMode=InputMotion  SensePosition=off  SenseVelocity=off  SenseAcceleration=off  SenseTorqueForce=on  SenseLowerLimitTorqueForce=off  SenseUpperLimitTorqueForce=off  LowerLimitSpecify=on  LowerLimitBound=range_ra_dip5_e_f(1)  LowerLimitBoundUnits=deg  LowerLimitStiffness=1e4  LowerLimitStiffnessUnits=N*m/deg  LowerLimitDamping=10  LowerLimitDampingUnits=N*m/(deg/s)  LowerLimitTransitionRegionWidth=0.1  LowerLimitTransitionRegionWidthUnits=deg  UpperLimitSpecify=on  UpperLimitBound=range_ra_dip5_e_f(2)  UpperLimitBoundUnits=deg  UpperLimitStiffness=1e4  UpperLimitStiffnessUnits=N*m/deg  UpperLimitDamping=10  UpperLimitDampingUnits=N*m/(deg/s)  UpperLimitTransitionRegionWidth=0.1  UpperLimitTransitionRegionWidthUnits=deg  PositionTargetSpecify=off  PositionTargetPriority=High  PositionTargetValue=ic_ra_dip5_e_f(1)  PositionTargetValueUnits=rad  VelocityTargetSpecify=off  VelocityTargetPriority=High  VelocityTargetValue=ic_ra_dip5_e_f(2)  VelocityTargetValueUnits=rad/s
  Rigid Transform : sm_lib/Frames and Transforms/Rigid Transform  TranslationMethod=None  TranslationStandardOffset=0  TranslationLengthUnit=m  TranslationStandardAxis=+Z  TranslationCartesianOffset=[0 0 0]  TranslationROffset=0  TranslationROffsetUnits=m  TranslationZOffset=0  TranslationZOffsetUnits=m  TranslationThetaOffset=0  TranslationThetaOffsetUnits=deg  RotationMethod=StandardAxis  RotationAngleUnits=deg  RotationStandardAxis=-Z  RotationAngle=180  RotationArbitraryAxis=[0 0 1]  FollAlignAxisA=+X  BaseAlignAxisA=+Y  FollAlignAxisB=+Y  BaseAlignAxisB=+Z  RotationSequenceAxes=FollowerAxes  RotationSequence=XYX  RotationSequenceAngles=[0 0 0]  RotationSequenceAnglesUnits=deg  RotationMatrix=[1 0 0; 0 1 0; 0 0 1]
  Simulink-PS Converter3 : nesl_utility/Simulink-PS Converter  PhysicalDomain=network_engine_domain  SubClassName=ps_input  LeftPortType=input  RightPortType=output  PseudoPeriodic=off  Frequencies=[]  NoiseDistribution=none  NoiseParameters=[]  Unit=rad  AffineConversion=on  FilteringAndDerivatives=provide  SimscapeFilterOrder=2  InputFilterTimeConstant=0.001  UdotUserProvided=2
  Conn1 : PMIOPort  Side=Left
  Conn2 : PMIOPort  Port=2  Side=Right
  Out1 : Outport  VectorParamsAs1DForOutWhenUnconnected=off
  wires:
  Demux3/1 -> Simulink-PS Converter3/1
  From Workspace3/1 -> Demux3/1
  Demux3/3 -> Simulink-PS Converter3/3
  PS-Simulink Converter/1 -> Out1/1  "MCP torque"
  Demux3/2 -> Simulink-PS Converter3/2
  connections:
  Simulink-PS Converter3/RConn1 -- Revolute Joint/LConn2
  PS-Simulink Converter/LConn1 -- Revolute Joint/RConn2
  Revolute Joint/RConn1 -- Conn2/RConn1
  Rigid Transform/LConn1 -- Conn1/RConn1
  Revolute Joint/LConn1 -- Rigid Transform/RConn1

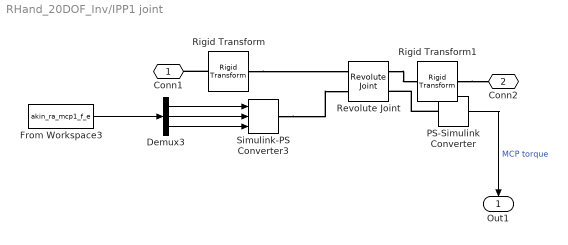
== system RHand_20DOF_Inv/IPP1 joint ==
  Demux3 : Demux  Outputs=3
  From Workspace3 : FromWorkspace  VariableName=akin_ra_mcp1_f_e  SampleTime=-1  OutputAfterFinalValue=Holding final value
  PS-Simulink Converter : nesl_utility/PS-Simulink Converter  PhysicalDomain=network_engine_domain  SubClassName=ps_output  LeftPortType=input  RightPortType=output  PseudoPeriodic=off  Frequencies=[]  Unit=N*m  AffineConversion=off
  Revolute Joint : sm_lib/Joints/Revolute Joint  JointMode=Normal  SenseConstraintForce=off  SenseConstraintForceX=off  SenseConstraintForceY=off  SenseConstraintForceZ=off  SenseConstraintTorque=off  SenseConstraintTorqueX=off  SenseConstraintTorqueY=off  SenseConstraintTorqueZ=off  SenseTotalForce=off  SenseTotalForceX=off  SenseTotalForceY=off  SenseTotalForceZ=off  SenseTotalTorque=off  SenseTotalTorqueX=off  SenseTotalTorqueY=off  SenseTotalTorqueZ=off  CompositeWrenchDir=FollowerOnBase  CompositeWrenchFrame=BaseFrame  EquilibriumPosition=dof_mech_ra_mcp1_f_e(1)  EquilibriumPositionUnits=rad  SpringStiffness=dof_mech_ra_mcp1_f_e(2)  SpringStiffnessUnits=N*m/rad  DampingCoefficient=dof_mech_ra_mcp1_f_e(3)  DampingCoefficientUnits=N*m/(rad/s)  TorqueActuationMode=ComputedTorque  MotionActuationMode=InputMotion  SensePosition=off  SenseVelocity=off  SenseAcceleration=off  SenseTorqueForce=on  SenseLowerLimitTorqueForce=off  SenseUpperLimitTorqueForce=off  LowerLimitSpecify=on  LowerLimitBound=range_ra_mcp1_f_e(1)  LowerLimitBoundUnits=deg  LowerLimitStiffness=1e4  LowerLimitStiffnessUnits=N*m/deg  LowerLimitDamping=10  LowerLimitDampingUnits=N*m/(deg/s)  LowerLimitTransitionRegionWidth=0.1  LowerLimitTransitionRegionWidthUnits=deg  UpperLimitSpecify=on  UpperLimitBound=range_ra_mcp1_f_e(2)  UpperLimitBoundUnits=deg  UpperLimitStiffness=1e4  UpperLimitStiffnessUnits=N*m/deg  UpperLimitDamping=10  UpperLimitDampingUnits=N*m/(deg/s)  UpperLimitTransitionRegionWidth=0.1  UpperLimitTransitionRegionWidthUnits=deg  PositionTargetSpecify=off  PositionTargetPriority=High  PositionTargetValue=ic_ra_mcp1_f_e(1)  PositionTargetValueUnits=rad  VelocityTargetSpecify=off  VelocityTargetPriority=High  VelocityTargetValue=ic_ra_mcp1_f_e(2)  VelocityTargetValueUnits=rad/s
  Rigid Transform : sm_lib/Frames and Transforms/Rigid Transform  TranslationMethod=None  TranslationStandardOffset=0  TranslationLengthUnit=m  TranslationStandardAxis=+Z  TranslationCartesianOffset=[0 0 0]  TranslationROffset=0  TranslationROffsetUnits=m  TranslationZOffset=0  TranslationZOffsetUnits=m  TranslationThetaOffset=0  TranslationThetaOffsetUnits=deg  RotationMethod=StandardAxis  RotationAngleUnits=deg  RotationStandardAxis=-X  RotationAngle=90  RotationArbitraryAxis=[0 0 1]  FollAlignAxisA=+X  BaseAlignAxisA=+Y  FollAlignAxisB=+Y  BaseAlignAxisB=+Z  RotationSequenceAxes=FollowerAxes  RotationSequence=XYX  RotationSequenceAngles=[0 0 0]  RotationSequenceAnglesUnits=deg  RotationMatrix=[1 0 0; 0 1 0; 0 0 1]
  Rigid Transform1 : sm_lib/Frames and Transforms/Rigid Transform  TranslationMethod=None  TranslationStandardOffset=0  TranslationLengthUnit=m  TranslationStandardAxis=+Z  TranslationCartesianOffset=[0 0 0]  TranslationROffset=0  TranslationROffsetUnits=m  TranslationZOffset=0  TranslationZOffsetUnits=m  TranslationThetaOffset=0  TranslationThetaOffsetUnits=deg  RotationMethod=StandardAxis  RotationAngleUnits=deg  RotationStandardAxis=+X  RotationAngle=90  RotationArbitraryAxis=[0 0 1]  FollAlignAxisA=+X  BaseAlignAxisA=+Y  FollAlignAxisB=+Y  BaseAlignAxisB=+Z  RotationSequenceAxes=FollowerAxes  RotationSequence=XYX  RotationSequenceAngles=[0 0 0]  RotationSequenceAnglesUnits=deg  RotationMatrix=[1 0 0; 0 1 0; 0 0 1]
  Simulink-PS Converter3 : nesl_utility/Simulink-PS Converter  PhysicalDomain=network_engine_domain  SubClassName=ps_input  LeftPortType=input  RightPortType=output  PseudoPeriodic=off  Frequencies=[]  NoiseDistribution=none  NoiseParameters=[]  Unit=rad  AffineConversion=on  FilteringAndDerivatives=provide  SimscapeFilterOrder=2  InputFilterTimeConstant=0.001  UdotUserProvided=2
  Conn1 : PMIOPort  Side=Left
  Conn2 : PMIOPort  Port=2  Side=Right
  Out1 : Outport  VectorParamsAs1DForOutWhenUnconnected=off
  wires:
  Demux3/1 -> Simulink-PS Converter3/1
  From Workspace3/1 -> Demux3/1
  Demux3/3 -> Simulink-PS Converter3/3
  PS-Simulink Converter/1 -> Out1/1  "MCP torque"
  Demux3/2 -> Simulink-PS Converter3/2
  connections:
  Simulink-PS Converter3/RConn1 -- Revolute Joint/LConn2
  PS-Simulink Converter/LConn1 -- Revolute Joint/RConn2
  Revolute Joint/RConn1 -- Rigid Transform1/LConn1
  Rigid Transform/LConn1 -- Conn1/RConn1
  Rigid Transform/RConn1 -- Revolute Joint/LConn1
  Rigid Transform1/RConn1 -- Conn2/RConn1

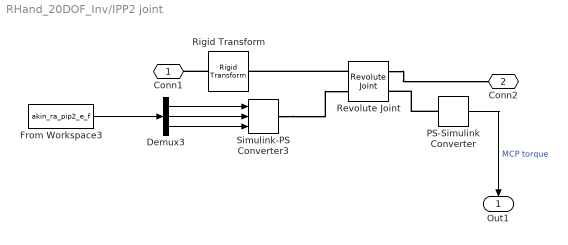
== system RHand_20DOF_Inv/IPP2 joint ==
  Demux3 : Demux  Outputs=3
  From Workspace3 : FromWorkspace  VariableName=akin_ra_pip2_e_f  SampleTime=-1  OutputAfterFinalValue=Holding final value
  PS-Simulink Converter : nesl_utility/PS-Simulink Converter  PhysicalDomain=network_engine_domain  SubClassName=ps_output  LeftPortType=input  RightPortType=output  PseudoPeriodic=off  Frequencies=[]  Unit=N*m  AffineConversion=off
  Revolute Joint : sm_lib/Joints/Revolute Joint  JointMode=Normal  SenseConstraintForce=off  SenseConstraintForceX=off  SenseConstraintForceY=off  SenseConstraintForceZ=off  SenseConstraintTorque=off  SenseConstraintTorqueX=off  SenseConstraintTorqueY=off  SenseConstraintTorqueZ=off  SenseTotalForce=off  SenseTotalForceX=off  SenseTotalForceY=off  SenseTotalForceZ=off  SenseTotalTorque=off  SenseTotalTorqueX=off  SenseTotalTorqueY=off  SenseTotalTorqueZ=off  CompositeWrenchDir=FollowerOnBase  CompositeWrenchFrame=BaseFrame  EquilibriumPosition=dof_mech_ra_pip2_e_f(1)  EquilibriumPositionUnits=rad  SpringStiffness=dof_mech_ra_pip2_e_f(2)  SpringStiffnessUnits=N*m/rad  DampingCoefficient=dof_mech_ra_pip2_e_f(3)  DampingCoefficientUnits=N*m/(rad/s)  TorqueActuationMode=ComputedTorque  MotionActuationMode=InputMotion  SensePosition=off  SenseVelocity=off  SenseAcceleration=off  SenseTorqueForce=on  SenseLowerLimitTorqueForce=off  SenseUpperLimitTorqueForce=off  LowerLimitSpecify=on  LowerLimitBound=range_ra_pip2_e_f(1)  LowerLimitBoundUnits=deg  LowerLimitStiffness=1e4  LowerLimitStiffnessUnits=N*m/deg  LowerLimitDamping=10  LowerLimitDampingUnits=N*m/(deg/s)  LowerLimitTransitionRegionWidth=0.1  LowerLimitTransitionRegionWidthUnits=deg  UpperLimitSpecify=on  UpperLimitBound=range_ra_pip2_e_f(2)  UpperLimitBoundUnits=deg  UpperLimitStiffness=1e4  UpperLimitStiffnessUnits=N*m/deg  UpperLimitDamping=10  UpperLimitDampingUnits=N*m/(deg/s)  UpperLimitTransitionRegionWidth=0.1  UpperLimitTransitionRegionWidthUnits=deg  PositionTargetSpecify=off  PositionTargetPriority=High  PositionTargetValue=ic_ra_pip2_e_f(1)  PositionTargetValueUnits=rad  VelocityTargetSpecify=off  VelocityTargetPriority=High  VelocityTargetValue=ic_ra_pip2_e_f(2)  VelocityTargetValueUnits=rad/s
  Rigid Transform : sm_lib/Frames and Transforms/Rigid Transform  TranslationMethod=None  TranslationStandardOffset=0  TranslationLengthUnit=m  TranslationStandardAxis=+Z  TranslationCartesianOffset=[0 0 0]  TranslationROffset=0  TranslationROffsetUnits=m  TranslationZOffset=0  TranslationZOffsetUnits=m  TranslationThetaOffset=0  TranslationThetaOffsetUnits=deg  RotationMethod=StandardAxis  RotationAngleUnits=deg  RotationStandardAxis=-Z  RotationAngle=180  RotationArbitraryAxis=[0 0 1]  FollAlignAxisA=+X  BaseAlignAxisA=+Y  FollAlignAxisB=+Y  BaseAlignAxisB=+Z  RotationSequenceAxes=FollowerAxes  RotationSequence=XYX  RotationSequenceAngles=[0 0 0]  RotationSequenceAnglesUnits=deg  RotationMatrix=[1 0 0; 0 1 0; 0 0 1]
  Simulink-PS Converter3 : nesl_utility/Simulink-PS Converter  PhysicalDomain=network_engine_domain  SubClassName=ps_input  LeftPortType=input  RightPortType=output  PseudoPeriodic=off  Frequencies=[]  NoiseDistribution=none  NoiseParameters=[]  Unit=rad  AffineConversion=on  FilteringAndDerivatives=provide  SimscapeFilterOrder=2  InputFilterTimeConstant=0.001  UdotUserProvided=2
  Conn1 : PMIOPort  Side=Left
  Conn2 : PMIOPort  Port=2  Side=Right
  Out1 : Outport  VectorParamsAs1DForOutWhenUnconnected=off
  wires:
  Demux3/1 -> Simulink-PS Converter3/1
  From Workspace3/1 -> Demux3/1
  Demux3/3 -> Simulink-PS Converter3/3
  PS-Simulink Converter/1 -> Out1/1  "MCP torque"
  Demux3/2 -> Simulink-PS Converter3/2
  connections:
  Simulink-PS Converter3/RConn1 -- Revolute Joint/LConn2
  PS-Simulink Converter/LConn1 -- Revolute Joint/RConn2
  Revolute Joint/RConn1 -- Conn2/RConn1
  Rigid Transform/LConn1 -- Conn1/RConn1
  Revolute Joint/LConn1 -- Rigid Transform/RConn1
